simulink model "Vereinfachte_Dehtellersteuerung"  (R2022a)
settings: Solver=ode3  StartTime=0.0  StopTime=10.0  FixedStep=0.01  RelTol=1e-3
values from neighbouring files (symbols this model uses):
  A = 5    [Parametriesierung.m]
  I = 0.5    [Parametriesierung.m]
  igetr = 1080    [Parametriesierung.m]
  K = 8    [Parametriesierung.m]
  MRK = 1    [Parametriesierung.m]
  PHI = 0.001    [Parametriesierung.m]
  Ra = 40    [Parametriesierung.m]
  U = 24    [Parametriesierung.m]
settings Model: Creator=60251  LastModifiedBy=60251

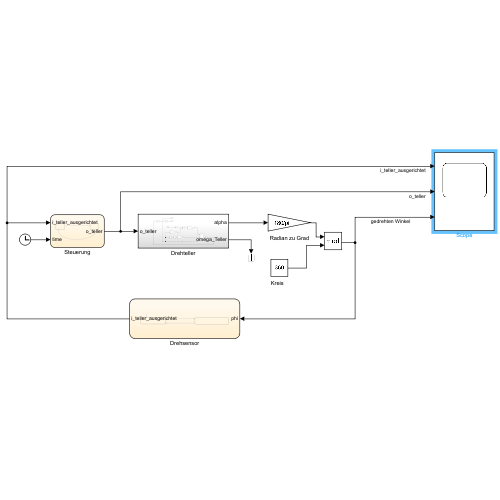
[thumbnail: Simulink's stored preview of the top-level diagram]
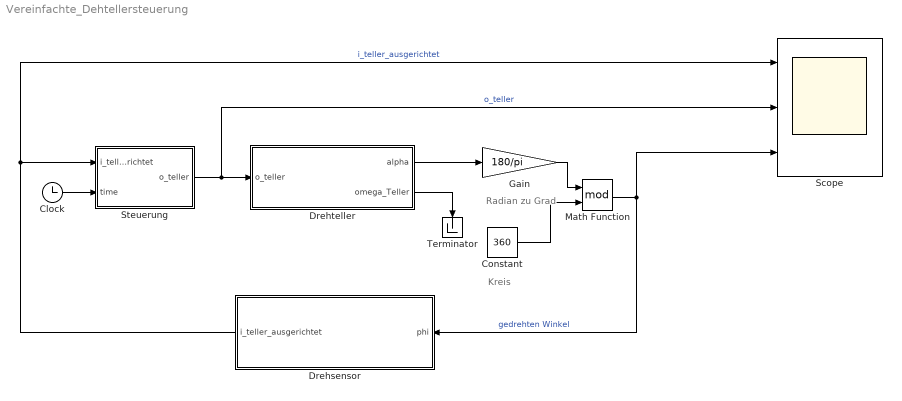
== system Vereinfachte_Dehtellersteuerung ==
  note: Kreis
  note: Radian zu Grad
  Clock : Clock
  Constant : Constant  Value=360
  Drehsensor : Stateflow chart  TreatAsAtomicUnit=on
  Drehteller : Subsystem
  Gain : Gain  Gain=180/pi
  Math Function : Math  Operator=mod
  Scope : Scope  NumInputPorts=3
  Steuerung : Stateflow chart  TreatAsAtomicUnit=on
  Terminator : Terminator
  wires:
  Steuerung/1(o_teller) -> Scope/2, Drehteller/1(o_teller)  "o_teller"
  Drehteller/1(alpha) -> Gain/1
  Drehteller/2(omega_Teller) -> Terminator/1
  Clock/1 -> Steuerung/2(time)
  Drehsensor/1(i_teller_ausgerichtet) -> Scope/1, Steuerung/1(i_teller_ausgerichtet)  "i_teller_ausgerichtet"
  Gain/1 -> Math Function/1
  Constant/1 -> Math Function/2
  Math Function/1 -> Scope/3, Drehsensor/1(phi)  "gedrehten Winkel"

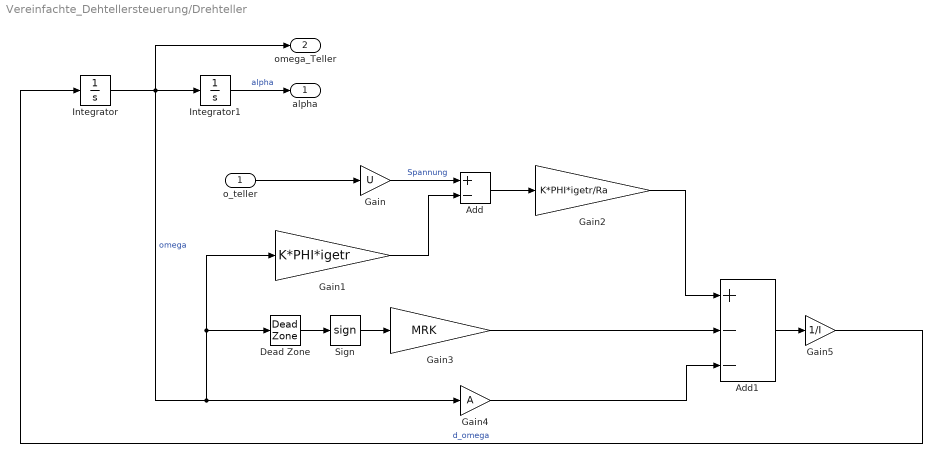
== system Vereinfachte_Dehtellersteuerung/Drehteller ==
  o_teller : Inport
  Add : Sum  Inputs=+-
  Add1 : Sum  Inputs=+--
  Dead Zone : DeadZone
  Gain : Gain  Gain=U
  Gain1 : Gain  Gain=K*PHI*igetr
  Gain2 : Gain  Gain=K*PHI*igetr/Ra
  Gain3 : Gain  Gain=MRK
  Gain4 : Gain  Gain=A
  Gain5 : Gain  Gain=1/I
  Integrator : Integrator
  Integrator1 : Integrator
  Sign : Signum
  alpha : Outport
  omega_Teller : Outport  Port=2
  wires:
  Add1/1 -> Gain5/1
  Integrator1/1 -> alpha/1  "alpha"
  Dead Zone/1 -> Sign/1
  Gain4/1 -> Add1/3
  Gain3/1 -> Add1/2
  Add/1 -> Gain2/1
  Sign/1 -> Gain3/1
  Gain5/1 -> Integrator/1  "d_omega"
  o_teller/1 -> Gain/1
  Gain/1 -> Add/1  "Spannung"
  Integrator/1 -> omega_Teller/1, Integrator1/1, Gain4/1, Gain1/1, Dead Zone/1  "omega"
  Gain1/1 -> Add/2
  Gain2/1 -> Add1/1

== stateflow chart Vereinfachte_Dehtellersteuerung/Drehsensor ==
  state eingerichtet
    en: i_teller_ausgerichtet = 0;
  state ausgerichtet
    en: i_teller_ausgerichtet = 1;
  (default) -> ausgerichtet
  ausgerichtet -> eingerichtet : [mod(phi+1, 90) > 2]
  eingerichtet -> ausgerichtet : [mod(phi+1, 90) <= 2]
  data: i_teller_ausgerichtet output; phi input

== stateflow chart Vereinfachte_Dehtellersteuerung/Steuerung ==
  state Motor_aus
    en: t = time;
    en: o_teller = 0;
  state Motor_an
    en: o_teller = 1;
    en: t = time;
  (default) -> Motor_aus
  Motor_aus -> Motor_an : [(time-t)>2]
  Motor_an -> Motor_aus : [i_teller_ausgerichtet==1 && (time-t)>0.5]
  data: i_teller_ausgerichtet input; o_teller output; time input; t local
